simulink model "Ch23_E01_bioreactor_mdl"  (Simulink 7.9)
settings: Solver=ode45  StartTime=0.0  StopTime=tstop  MaxStep=0.1  RelTol=1e-3
values from neighbouring files (symbols this model uses):
  D = 0.05:.05:0.5    [Ch01_Matlab_Tips.m]    (also in Ch04_PredatorPrey.m = jacobian(@(u)g(xss,u),0); Ch08_Bioreactor_Continuous.m = @(t,x) max(0, 0.1 + Kp*(Sp(t) - x(2)) + Ki*x(4)); Ch12_PID.m = Kp*tf([Td 0],[Td/N 1],'TimeUnit','minutes'); Ch12_PID_2DOF.m = @(Td) tf([Td 0],[Td/10 1],'TimeUnit','minutes'))
  deriv = @(cA,T,Tc) [      (q/V)*(cAi - cA) - k(T)*cA ... (first row only)    [Ch02_E05_CSTR.m]    (also in Ch02_Lorenz.m = @(t,x) [      -sig*x(1) + sig*x(2);      rho*x(1) - x(2) - x; Ch02_Lorenz_chebfun.m = @(t,x) [      -sig*x(1) + sig*x(2);      rho*x(1) - x(2) - x; Ch04_PredatorPrey.m = @(x) [dH(x(1),x(2)); dL(x(1),x(2))]; Ch04_PredatorPrey_chebfun.m = @(x) [dH(x(1),x(2)); dL(x(1),x(2))])
  x0 = [20;20]    [Ch01_Matlab_Tips.m]    (also in Ch23_E01_bioreactor copy.m = trim(mdl); Ch23_E01_bioreactor.m = trim(mdl); Ch23_E01_bioreactor_PID.m = xss_1; Ch24_CircadianClock.m = [M0;P0])
libraries: simulink x1
settings Model: Creator=jeff  LastModifiedBy=jeff

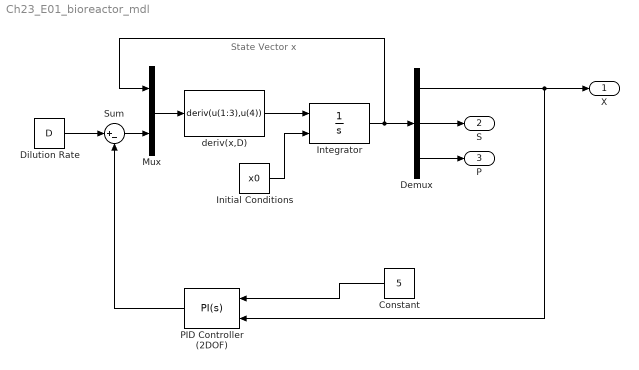
== system Ch23_E01_bioreactor_mdl ==
  note: State Vector x
  Constant : Constant  Value=5
  Demux : Demux  Outputs=3
  "Dilution Rate " : Constant  Value=D
  Initial Conditions : Constant  Value=x0  VectorParams1D=off
  Integrator : Integrator  InitialConditionSource=external  InitialCondition=x0  ContinuousStateAttributes={'X','S','P'}
  Mux : Mux  Inputs=2
  PID Controller (2DOF) : simulink/Continuous/PID Controller (2DOF)  Controller=PI  TimeDomain=Continuous-time  SampleTime=1  IntegratorMethod=Forward Euler  FilterMethod=Forward Euler  Form=Parallel  P=0  I=0.0020483758105338  D=-0.187537701233975  N=186.814439548907  b=1  c=1  InitialConditionSource=internal  InitialConditionForIntegrator=0  InitialConditionForFilter=0  ExternalReset=none  LimitOutput=off  UpperSaturationLimit=inf  LowerSaturationLimit=-inf  LinearizeAsGain=off  AntiWindupMode=none  Kb=1  TrackingMode=off  Kt=1  PParamMin=[]  PParamMax=[]  IParamMin=[]  IParamMax=[]  DParamMin=[]  DParamMax=[]  NParamMin=[]  NParamMax=[]  bParamMin=[]  bParamMax=[]  cParamMin=[]  cParamMax=[]  KbParamMin=[]  KbParamMax=[]  KtParamMin=[]  KtParamMax=[]  POutMin=[]  POutMax=[]  IOutMin=[]  IOutMax=[]  DOutMin=[]  DOutMax=[]  NOutMin=[]  NOutMax=[]  bOutMin=[]  bOutMax=[]  cOutMin=[]  cOutMax=[]  KbOutMin=[]  KbOutMax=[]  KtOutMin=[]  KtOutMax=[]  IntegratorOutMin=[]  IntegratorOutMax=[]  FilterOutMin=[]  FilterOutMax=[]  SumOutMin=[]  SumOutMax=[]  Sum1OutMin=[]  Sum1OutMax=[]  Sum2OutMin=[]  Sum2OutMax=[]  Sum3OutMin=[]  Sum3OutMax=[]  SumI1OutMin=[]  SumI1OutMax=[]  SumI2OutMin=[]  SumI2OutMax=[]  SumI3OutMin=[]  SumI3OutMax=[]  SumDOutMin=[]  SumDOutMax=[]  SaturationOutMin=[]  SaturationOutMax=[]  IntegratorContinuousStateAttributes=''  IntegratorStateMustResolveToSignalObject=off  IntegratorRTWStateStorageClass=Auto  FilterContinuousStateAttributes=''  FilterStateMustResolveToSignalObject=off  FilterRTWStateStorageClass=Auto
  Sum : Sum  Inputs=|+-
  deriv(x,D) : MATLABFcn  MATLABFcn=deriv(u(1:3),u(4))
  X : Outport
  S : Outport  Port=2
  P : Outport  Port=3
  wires:
  Initial Conditions/1 -> Integrator/2
  Mux/1 -> deriv(x,D)/1
  Integrator/1 -> Mux/1, Demux/1
  deriv(x,D)/1 -> Integrator/1
  Demux/1 -> X/1, PID Controller (2DOF)/2
  Demux/2 -> S/1
  Demux/3 -> P/1
  Constant/1 -> PID Controller (2DOF)/1
  "Dilution Rate "/1 -> Sum/1
  Sum/1 -> Mux/2
  PID Controller (2DOF)/1 -> Sum/2
